simulink model "simLeo"  (R2015a)
settings: Solver=ode45  StartTime=0.0  StopTime=10  RelTol=1e-3
settings Model: Creator=user  LastModifiedBy=user

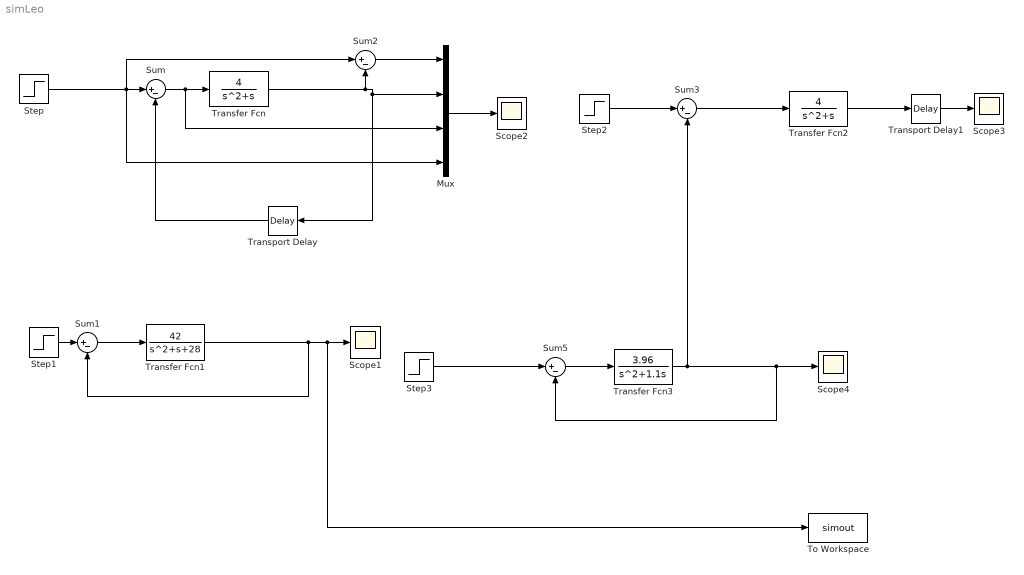
== system simLeo ==
  Mux : Mux
  Scope{1..4} (4 alike) : Scope
      Scope2 settings: YMin=-20  YMax=20  SaveName=ScopeData2
      Scope4 settings: SaveName=ScopeData3
  Step : Step  Time=0  SampleTime=0
  Step1 : Step  Time=0  After=900  SampleTime=0
  Step2 : Step  Time=0  SampleTime=0
  Step3 : Step  Time=0  SampleTime=0
  Sum{,1..3,5} (5 alike) : Sum  Inputs=|+-
  To Workspace : ToWorkspace  VariableName=simout  SaveFormat=Timeseries  SampleTime=-1
  Transfer Fcn : TransferFcn  Numerator=[4]  Denominator=[1 1 0]
  Transfer Fcn1 : TransferFcn  Numerator=[42]  Denominator=[1 1 28]
  Transfer Fcn2 : TransferFcn  Numerator=[4]  Denominator=[1 1 0]
  Transfer Fcn3 : TransferFcn  Numerator=[3.96]  Denominator=[1 1.1 0]
  Transport Delay : TransportDelay
  Transport Delay1 : TransportDelay
  wires:
  Transfer Fcn/1 -> Transport Delay/1, Mux/2, Sum2/2
  Sum/1 -> Mux/3, Transfer Fcn/1
  Step/1 -> Mux/4, Sum2/1, Sum/1
  Transfer Fcn1/1 -> To Workspace/1, Scope1/1, Sum1/2
  Sum1/1 -> Transfer Fcn1/1
  Step1/1 -> Sum1/1
  Transport Delay/1 -> Sum/2
  Mux/1 -> Scope2/1
  Sum2/1 -> Mux/1
  Transfer Fcn2/1 -> Transport Delay1/1
  Sum3/1 -> Transfer Fcn2/1
  Transfer Fcn3/1 -> Scope4/1, Sum5/2, Sum3/2
  Sum5/1 -> Transfer Fcn3/1
  Step3/1 -> Sum5/1
  Step2/1 -> Sum3/1
  Transport Delay1/1 -> Scope3/1
